simulink model "dist2"  (R2025b)
settings: Solver=FixedStepDiscrete  StartTime=0.0  StopTime=inf  FixedStep=128/48000  RelTol=1e-3
model workspace (MATLAB code in the model file):
  | Gain_rt = Simulink.Parameter(1.0);
  | Bypass_rt = Simulink.Parameter(false);
undefined symbols (not defined in the file): Amount_rt, Asym_rt, Attack_rt, Level_rt, Mix_rt, Release_rt, Shaper_rt, Tone_rt
settings Model: Creator=linogarciamorales  LastModifiedBy=linogarciamorales
settings OptimizationCC: EnhancedBackFolding=on  PassReuseOutputArgsAs=Individual arguments  ZeroExternalMemoryAtStartup=off  ZeroInternalMemoryAtStartup=off  OptimizeBlockOrder=speed  DifferentSizesBufferReuse=on  OptimizationCustomize=off  EfficientTunableParamExpr=on
settings DebuggingCC: ParameterTunabilityLossMsg=error
settings SFSimCC: MATLABDynamicMemAlloc=off
settings RTWCC: SystemTargetFile=ert.tlc  GenCodeOnly=on  TemplateMakefile=ert_default_tmf  Description=Embedded Coder
settings CodeAppCC: ForceParamTrailComments=on  IgnoreCustomStorageClasses=off  OperatorAnnotations=on  SimulinkDataObjDesc=on  SFDataObjDesc=on  InsertBlockDesc=on
settings ERTTargetCC: InlinedParameterPlacement=Hierarchical  ERTCustomFileTemplate=example_file_process.tlc  TargetLangStandard=C99 (ISO)  GenerateSampleERTMain=on  SupportNonInlinedSFcns=on

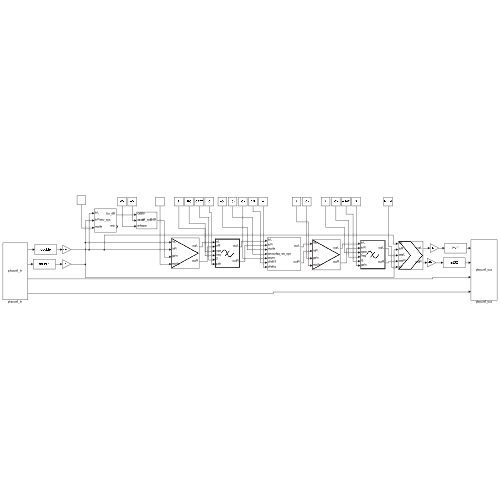
[thumbnail: Simulink's stored preview of the top-level diagram]
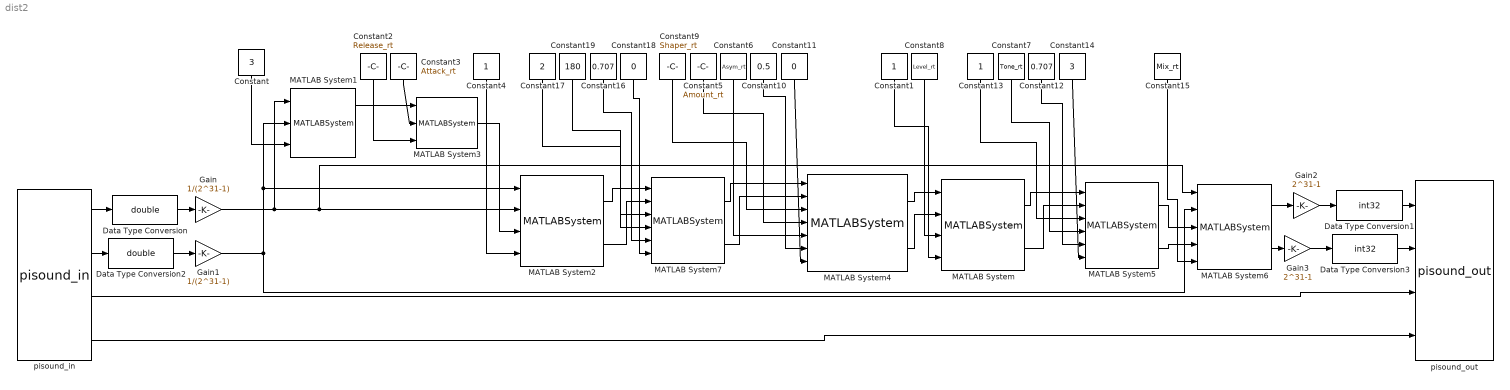
== system dist2 ==
  Constant : Constant  Value=3  OutDataTypeStr=uint8
  Constant1 : Constant  OutDataTypeStr=uint8
  Constant10 : Constant  Value=0.5  OutDataTypeStr=double
  Constant11 : Constant  Value=0  OutDataTypeStr=double
  Constant12 : Constant  Value=0.707  OutDataTypeStr=double
  Constant13 : Constant  OutDataTypeStr=uint8
  Constant14 : Constant  Value=3  OutDataTypeStr=double
  Constant15 : Constant  Value=Mix_rt  OutDataTypeStr=double
  Constant16 : Constant  Value=0.707  OutDataTypeStr=double
  Constant17 : Constant  Value=2  OutDataTypeStr=uint8
  Constant18 : Constant  Value=0  OutDataTypeStr=double
  Constant19 : Constant  Value=180  OutDataTypeStr=double
  Constant2 : Constant  Value=Release_rt  OutDataTypeStr=double
  Constant3 : Constant  Value=Attack_rt  OutDataTypeStr=double
  Constant4 : Constant  OutDataTypeStr=uint8
  Constant5 : Constant  Value=Amount_rt  OutDataTypeStr=double
  Constant6 : Constant  Value=Asym_rt  OutDataTypeStr=double
  Constant7 : Constant  Value=Tone_rt  OutDataTypeStr=double
  Constant8 : Constant  Value=Level_rt  OutDataTypeStr=double
  Constant9 : Constant  Value=Shaper_rt  OutDataTypeStr=uint8
  Data Type Conversion : DataTypeConversion  OutDataTypeStr=double  SaturateOnIntegerOverflow=off  RndMeth=Floor
  Data Type Conversion1 : DataTypeConversion  OutDataTypeStr=int32  SaturateOnIntegerOverflow=off  RndMeth=Floor
  Data Type Conversion2 : DataTypeConversion  OutDataTypeStr=double  SaturateOnIntegerOverflow=off  RndMeth=Floor
  Data Type Conversion3 : DataTypeConversion  OutDataTypeStr=int32  SaturateOnIntegerOverflow=off  RndMeth=Floor
  Gain : Gain  Gain=1/(2^31-1)
  Gain1 : Gain  Gain=1/(2^31-1)
  Gain2 : Gain  Gain=2^31-1
  Gain3 : Gain  Gain=2^31-1
  MATLAB System : MATLABSystem  System=vca_sys  N=128  Fs=48000  bypass=uint8(0)  SimulateUsing=Code generation
      mask Type: vca_sys
  MATLAB System1 : MATLABSystem  System=env_sys  N=128  Fs=48000  ModeDefault=uint8( 1 )  Eps=1e-12  TauRMS=0.015  SimulateUsing=Code generation
      mask Type: env_sys
  MATLAB System2 : MATLABSystem  System=vca_sys  N=128  Fs=48000  bypass=uint8(0)  SimulateUsing=Code generation
      mask Type: vca_sys
  MATLAB System3 : MATLABSystem  System=arf_sys  N=128  Fs=48000  AttackDefault=0.010  ReleaseDefault=0.100  SimulateUsing=Code generation
      mask Type: arf_sys
  MATLAB System4 : MATLABSystem  System=lut_ws_sys  N=128  M=257  bypass=uint8(0)  ModeDefault=uint8( 3 )  AmountDefault=12.0  AsymDefault=0.0  Cheb3Default=1.0  Cheb5Default=0.0  XUser=linspace( -1, 1, 257 )  YUser=linspace( -1, 1, 257 )  MUser=257  Eps=1e-12  SimulateUsing=Code generation
      mask Type: lut_ws_sys
  MATLAB System5 : MATLABSystem  System=vcf_sys  N=128  Fs=48000  bypass=uint8(0)  SimulateUsing=Code generation
      mask Type: vcf_sys
  MATLAB System6 : MATLABSystem  System=mix_sys  N=128  Fs=48000  Mode=uint8( 0 )  SmoothTime=0.01  IndepInDB=false  SimulateUsing=Code generation
      mask Type: mix_sys
  MATLAB System7 : MATLABSystem  System=vcf_sys  N=128  Fs=48000  bypass=uint8(0)  SimulateUsing=Code generation
      mask Type: vcf_sys
  pisound_in : S-Function  FunctionName=pisound_in  Parameters=48000, 128, 0  SFunctionDeploymentMode=off  EnableBusSupport=off
  pisound_out : S-Function  FunctionName=pisound_out  Parameters=48000, 128, 0  SFunctionDeploymentMode=off  EnableBusSupport=off
  wires:
  pisound_in/1 -> Data Type Conversion/1
  pisound_in/2 -> Data Type Conversion2/1
  Data Type Conversion1/1 -> pisound_out/1
  Data Type Conversion3/1 -> pisound_out/2
  Gain2/1 -> Data Type Conversion1/1
  Gain3/1 -> Data Type Conversion3/1
  Data Type Conversion/1 -> Gain/1
  Data Type Conversion2/1 -> Gain1/1
  pisound_in/3 -> pisound_out/3
  pisound_in/4 -> pisound_out/4
  Gain/1 -> MATLAB System2/2, MATLAB System6/1, MATLAB System1/1
  Gain1/1 -> MATLAB System6/2, MATLAB System1/2, MATLAB System2/1
  Constant/1 -> MATLAB System1/3
  Constant1/1 -> MATLAB System/4
  Constant2/1 -> MATLAB System3/3
  Constant3/1 -> MATLAB System3/2
  MATLAB System3/1 -> MATLAB System2/3
  MATLAB System4/1 -> MATLAB System/1
  MATLAB System4/2 -> MATLAB System/2
  Constant8/1 -> MATLAB System/3
  Constant9/1 -> MATLAB System4/3
  Constant5/1 -> MATLAB System4/4
  Constant6/1 -> MATLAB System4/5
  Constant7/1 -> MATLAB System5/4
  MATLAB System/1 -> MATLAB System5/1
  MATLAB System/2 -> MATLAB System5/2
  MATLAB System1/1 -> MATLAB System3/1
  Constant4/1 -> MATLAB System2/4
  Constant10/1 -> MATLAB System4/6
  Constant11/1 -> MATLAB System4/7
  Constant12/1 -> MATLAB System5/5
  Constant13/1 -> MATLAB System5/3
  Constant14/1 -> MATLAB System5/6
  MATLAB System6/1 -> Gain2/1
  MATLAB System6/2 -> Gain3/1
  MATLAB System5/1 -> MATLAB System6/3
  MATLAB System5/2 -> MATLAB System6/4
  Constant15/1 -> MATLAB System6/5
  Constant19/1 -> MATLAB System7/4
  Constant17/1 -> MATLAB System7/3
  Constant16/1 -> MATLAB System7/5
  Constant18/1 -> MATLAB System7/6
  MATLAB System2/1 -> MATLAB System7/1
  MATLAB System2/2 -> MATLAB System7/2
  MATLAB System7/1 -> MATLAB System4/1
  MATLAB System7/2 -> MATLAB System4/2
